simulink model "InverterTestSystemMotorSettings_168_124"  (R2020a)
settings: Solver=ode4  StartTime=0.0  StopTime=inf  FixedStep=Ts  RelTol=1e-3  EnableMultiTasking=on
values from neighbouring files (symbols this model uses):
  SimulinkOutputBusChannelCount = c    [ITS_Create_Simulation_Interface_Buses.m]
undefined symbols (not defined in the file or in its folder): DiscIntNeverNeededParam, signal1, signal2, signal3, signal4, signal5, signal6, signal7
settings Model: SimulationMode=external  ExtModeTrigDuration=16000  ExtModeTrigLevel=10  Creator=Vincent  LastModifiedBy=maccl
settings SolverCC: PositivePriorityOrder=on  AutoInsertRateTranBlk=on  InsertRTBMode=Always
settings DataIOCC: LimitDataPoints=on  MaxDataPoints=200000  SaveFormat=Array  SaveOutput=off  SignalLogging=off  DSMLogging=off  SaveTime=off  ReturnWorkspaceOutputs=off
settings OptimizationCC: EnhancedBackFolding=on  PassReuseOutputArgsThreshold=0  ExpressionDepthLimit=2147483647  LifeSpan=1095  MaxStackSize=64  OptimizeBlockOrder=speed  DifferentSizesBufferReuse=on  OptimizationCustomize=off
settings DebuggingCC: UnderspecifiedInitializationDetection=Classic  MergeDetectMultiDrivingBlocksExec=none  SolverPrmCheckMsg=warning  ParameterTunabilityLossMsg=error  BusObjectLabelMismatch=none  StateNameClashWarn=warning  SFUnexpectedBacktrackingDiag=warning  SFNoUnconditionalDefaultTransitionDiag=warning  SFExecutionAtInitializationDiag=none  ArithmeticOperatorsInVariantConditions=warning
settings HardwareCC: ProdBitPerLong=64  ProdHWDeviceType=Intel->x86-64 (Linux 64)  TargetHWDeviceType=32-bit Generic
settings SFSimCC: SimUseLocalCustomCode=off  CustomCodeUndefinedFunction=UseInterfaceOnly
settings RTWCC: Description=slxrt NI Linux Real-Time x86_64 Targets  SystemTargetFile=ni_slxrt.tlc  PackageName=main_code.zip  GenerateReport=on  RTWUseLocalCustomCode=off  Toolchain=GCC Compiler for VeriStand NI Linux Real-Time targets | gmake makefile (64-bit Windows)  BuildConfiguration=Faster Runs  LaunchReport=on
settings CodeAppCC: ForceParamTrailComments=on  OperatorAnnotations=on  MATLABSourceComments=on
settings STFCustomTargetCC: UseToolchainInfoCompliant=on  SystemTargetFile=ni_slxrt.tlc
settings GRTTargetCC: TargetLangStandard=C89/C90 (ANSI)  ParMdlRefBuildCompliant=off  CompOptLevelCompliant=off  ConcurrentExecutionCompliant=off  CombineOutputUpdateFcns=off  MatFileLogging=off  CPPClassGenCompliant=off  ExtMode=on  ExtModeMexArgs='10.0.35.12',0,17725  RTWCAPISignals=on  RTWCAPIParams=on  RTWCAPIStates=on  RTWCAPIRootIO=on
settings ConfigComp: CovMetricSettings=dw  CovHtmlReporting=on  CovSaveCumulativeToWorkspaceVar=on  CovSaveSingleToWorkspaceVar=on  CovExternalEMLEnable=off

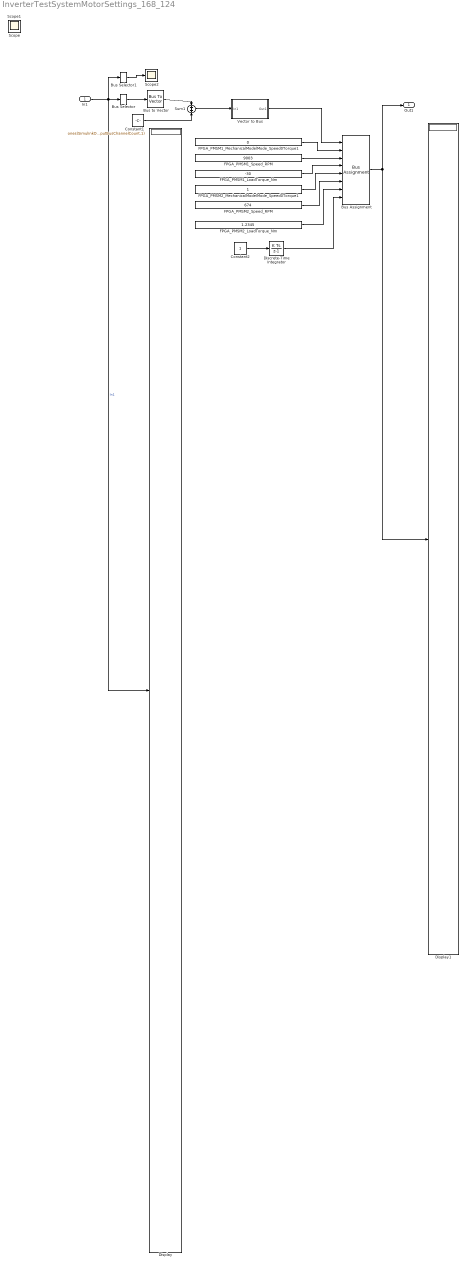
== system InverterTestSystemMotorSettings_168_124 ==
  In1 : Inport  OutDataTypeStr=Bus: SimulinkInputBus
  Bus Assignment : BusAssignment  AssignedSignals=signal1,signal2,signal3,signal4,signal5,signal6,signal7
  Bus Selector : BusSelector  OutputSignals=In001_PMSM1_CurrentPhaseA_A,In002_PMSM1_CurrentPhaseB_A,In003_PMSM1_CurrentPhaseC_A,In004_PMSM1_VoltageAveragePhaseA_V,In005_PMSM1_VoltageAveragePhaseB_V,In006_PMSM1_VoltageAveragePhaseC_V,In007_PMSM1_ThreePhaseActivePower_W,In008_PMSM1_ThreePhaseReactivePower_VAR,In009_PMSM1_DirectStatorCurrentId_A,In010_PMSM1_QuadratureStatorCurrentIq_A,In011_PMSM1_MechanicalAngle_deg,In012_PMSM1_ElectricalAngle_deg,In013_PMSM1_Torque_Nm,In014_PMSM1_ResolverSine,In015_PMSM1_ResolverCosine,In016_PMSM1_ResolverCarrier,In017_PMSM1_ResolverAngle_deg,In018_PMSM1_Speed_RPM,In019_PMSM1_TotalTorque_Nm,In020_PMSM1_BackEMFPhaseA_V,In021_PMSM1_BackEMFPhaseB_V,In022_PMSM1_BackEMFPhaseC_V,In023_PMSM2_CurrentPhaseA_A,In024_PMSM2_CurrentPhaseB_A,In025_PMSM2_CurrentPhaseC_A,In026_PMSM2_VoltageAveragePhaseA_V,In027_PMSM2_VoltageAveragePhaseB_V,In028_PMSM2_VoltageAveragePhaseC_V,In029_PMSM2_ThreePhaseActivePower_W,In030_PMSM2_ThreePhaseReactivePower_VAR,In031_PMSM2_DirectStatorCurrentId_A,In032_PMSM2_QuadratureStatorCurrentIq_A,In033_PMSM2_MechanicalAngle_deg,In034_PMSM2_ElectricalAngle_deg,In035_PMSM2_Torque_Nm,In036_PMSM2_ResolverSine,In037_PMSM2_ResolverCosine,In038_PMSM2_ResolverCarrier,In039_PMSM2_ResolverAngle_deg,In040_PMSM2_Speed_RPM,In041_PMSM2_TotalTorque_Nm,In042_PMSM2_BackEMFPhaseA_V,In043_PMSM2_BackEMFPhaseB_V,In044_PMSM2_BackEMFPhaseC_V,In045_Measurements_001,In046_Measurements_002,In047_Measurements_003,In048_Measurements_004,In049_Measurements_005,In050_Measurements_006,In051_Measurements_007,In052_Measurements_008,In053_Measurements_009,In054_Measurements_010,In055_Measurements_011,In056_Measurements_012,In057_Measurements_013,In058_Measurements_014,In059_Measurements_015,In060_Measurements_016,In061_Measurements_017,In062_Measurements_018,In063_Measurements_019,In064_Measurements_020,In065_Measurements_021,In066_Measurements_022,In067_Measurements_023,In068_Measurements_024,In069_Measurements_025,In070_Measurements_026,In071_Measurements_027,In072_Measurements_028,In073_Measurements_029,In074_Measurements_030,In075_Measurements_031,In076_Measurements_032,In077_Measurements_033,In078_Measurements_034,In079_Measurements_035,In080_Measurements_036,In081_Measurements_037,In082_Measurements_038,In083_Measurements_039,In084_Measurements_040,In085_Measurements_041,In086_Measurements_042,In087_Measurements_043,In088_Measurements_044,In089_Measurements_045,In090_Measurements_046,In091_Measurements_047,In092_Measurements_048,In093_Measurements_049,In094_Measurements_050,In095_Measurements_051,In096_Measurements_052,In097_Measurements_053,In098_Measurements_054,In099_Measurements_055,In100_Measurements_056,In101_Measurements_057,In102_Measurements_058,In103_Measurements_059,In104_Measurements_060,In105_Measurements_061,In106_Measurements_062,In107_Measurements_063,In108_Measurements_064,In109_AnalogOutputs_001,In110_AnalogOutputs_002,In111_AnalogOutputs_003,In112_AnalogOutputs_004,In113_AnalogOutputs_005,In114_AnalogOutputs_006,In115_AnalogOutputs_007,In116_AnalogOutputs_008,In117_AnalogOutputs_009,In118_AnalogOutputs_010,In119_AnalogOutputs_011,In120_AnalogOutputs_012,In121_AnalogOutputs_013,In122_AnalogOutputs_014,In123_AnalogOutputs_015,In124_AnalogOutputs_016  OutputAsBus=on
  Bus Selector1 : BusSelector  OutputSignals=In001_PMSM1_CurrentPhaseA_A,In002_PMSM1_CurrentPhaseB_A,In003_PMSM1_CurrentPhaseC_A  OutputAsBus=on
  Bus to Vector : BusToVector
  Constant1 : Constant  Value=ones(SimulinkOutputBusChannelCount,1)  SampleTime=-1
  Constant2 : Constant  SampleTime=-1
  Discrete-Time Integrator : DiscreteIntegrator  SampleTime=-1  ICPrevOutput=DiscIntNeverNeededParam  ICPrevScaledInput=DiscIntNeverNeededParam
  Display : Display
  Display1 : Display
  FPGA_PMSM1_LoadTorque_Nm : Constant  Value=-30  SampleTime=-1
  FPGA_PMSM1_MechanicalModelMode_Speed0Torque1 : Constant  Value=0  SampleTime=-1
  FPGA_PMSM1_Speed_RPM : Constant  Value=9003  SampleTime=-1
  FPGA_PMSM2_LoadTorque_Nm : Constant  Value=1.2345  SampleTime=-1
  FPGA_PMSM2_MechanicalModelMode_Speed0Torque1 : Constant  SampleTime=-1
  FPGA_PMSM2_Speed_RPM : Constant  Value=674  SampleTime=-1
  Scope2 : Scope
  Sum1 : Sum
  Vector to Bus : Subsystem  mask{Nsigs=SimulinkOutputBusChannelCount}
      mask prompts: Nsigs "Signal Length"
      mask init:
      | CurrentSys = gcs;
      | blockName = get_param(gcb,'Name');
      | oldNsigs = str2num(get_param([CurrentSys '/' blockName '/Demux'],'Outputs'));
      | newNsigs = str2num(get_param([CurrentSys '/' blockName], 'Nsigs'));
      | 
      | if newNsigs > oldNsigs,
      |     set_param([CurrentSys '/' blockName '/Demux'],'Outputs',num2str(newNsigs))
      |     set_param([CurrentSys '/' blockName '/BusCreator'],'Inputs',num2str(newNsigs))
      |     for nnn = (oldNsigs+1):newNsigs,
      |         add_line([CurrentSys '/' blockName],['Demux/' num2str(nnn)],['BusCreator/' num2str(nnn)])
      |     end
      | elseif newNsigs < oldNsigs,
      |     for nnn = (newNsigs+1):oldNsigs,
      |         delete_line([CurrentSys '/' blockName],['Demux/' num2str(nnn)],['BusCreator/' num2str(nnn)])
      |     end
      |     set_param([CurrentSys '/' blockName '/Demux'],'Outputs',num2str(newNsigs))
      |     set_param([CurrentSys '/' blockName '/BusCreator'],'Inputs',num2str(newNsigs))
      | end
  Out1 : Outport  SignalName=Out1  OutDataTypeStr=Bus: SimulinkOutputBus  VectorParamsAs1DForOutWhenUnconnected=off
  Scope : Scope
  Scope1 : Scope
  wires:
  In1/1 -> Bus Selector1/1, Bus Selector/1, Display/1  "In1"
  Constant1/1 -> Sum1/2
  Bus to Vector/1 -> Sum1/1
  Sum1/1 -> Vector to Bus/1(In1)
  Bus Selector/1 -> Bus to Vector/1
  Vector to Bus/1(Out1) -> Bus Assignment/1
  Bus Assignment/1 -> Out1/1, Display1/1
  FPGA_PMSM1_MechanicalModelMode_Speed0Torque1/1 -> Bus Assignment/2
  FPGA_PMSM1_Speed_RPM/1 -> Bus Assignment/3
  FPGA_PMSM1_LoadTorque_Nm/1 -> Bus Assignment/4
  FPGA_PMSM2_MechanicalModelMode_Speed0Torque1/1 -> Bus Assignment/5
  FPGA_PMSM2_Speed_RPM/1 -> Bus Assignment/6
  FPGA_PMSM2_LoadTorque_Nm/1 -> Bus Assignment/7
  Constant2/1 -> Discrete-Time Integrator/1
  Discrete-Time Integrator/1 -> Bus Assignment/8
  Bus Selector1/1 -> Scope2/1

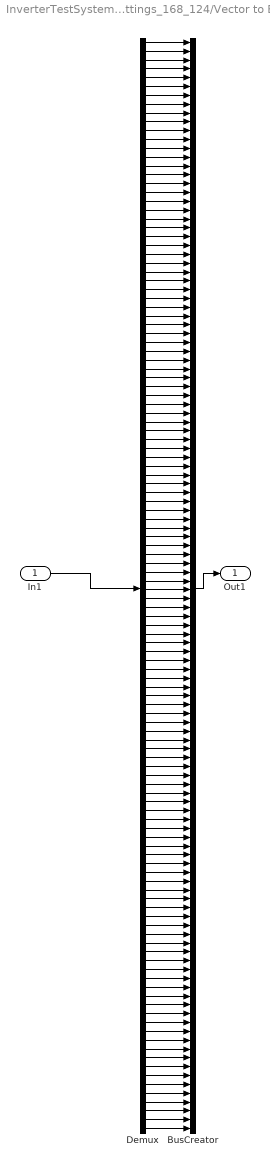
== system InverterTestSystemMotorSettings_168_124/Vector to Bus ==
  In1 : Inport
  BusCreator : BusCreator  Inputs=124
  Demux : Demux  Outputs=124
  Out1 : Outport  VectorParamsAs1DForOutWhenUnconnected=off
  wires:
  Demux/7 -> BusCreator/7
  Demux/6 -> BusCreator/6
  Demux/5 -> BusCreator/5
  Demux/1 -> BusCreator/1
  Demux/2 -> BusCreator/2
  BusCreator/1 -> Out1/1
  In1/1 -> Demux/1
  Demux/3 -> BusCreator/3
  Demux/4 -> BusCreator/4
  Demux/8 -> BusCreator/8
  Demux/9 -> BusCreator/9
  Demux/10 -> BusCreator/10
  Demux/11 -> BusCreator/11
  Demux/12 -> BusCreator/12
  Demux/13 -> BusCreator/13
  Demux/14 -> BusCreator/14
  Demux/15 -> BusCreator/15
  Demux/16 -> BusCreator/16
  Demux/17 -> BusCreator/17
  Demux/18 -> BusCreator/18
  Demux/19 -> BusCreator/19
  Demux/20 -> BusCreator/20
  Demux/21 -> BusCreator/21
  Demux/22 -> BusCreator/22
  Demux/23 -> BusCreator/23
  Demux/24 -> BusCreator/24
  Demux/25 -> BusCreator/25
  Demux/26 -> BusCreator/26
  Demux/27 -> BusCreator/27
  Demux/28 -> BusCreator/28
  Demux/29 -> BusCreator/29
  Demux/30 -> BusCreator/30
  Demux/31 -> BusCreator/31
  Demux/32 -> BusCreator/32
  Demux/33 -> BusCreator/33
  Demux/34 -> BusCreator/34
  Demux/35 -> BusCreator/35
  Demux/36 -> BusCreator/36
  Demux/37 -> BusCreator/37
  Demux/38 -> BusCreator/38
  Demux/39 -> BusCreator/39
  Demux/40 -> BusCreator/40
  Demux/41 -> BusCreator/41
  Demux/42 -> BusCreator/42
  Demux/43 -> BusCreator/43
  Demux/44 -> BusCreator/44
  Demux/45 -> BusCreator/45
  Demux/46 -> BusCreator/46
  Demux/47 -> BusCreator/47
  Demux/48 -> BusCreator/48
  Demux/49 -> BusCreator/49
  Demux/50 -> BusCreator/50
  Demux/51 -> BusCreator/51
  Demux/52 -> BusCreator/52
  Demux/53 -> BusCreator/53
  Demux/54 -> BusCreator/54
  Demux/55 -> BusCreator/55
  Demux/56 -> BusCreator/56
  Demux/57 -> BusCreator/57
  Demux/58 -> BusCreator/58
  Demux/59 -> BusCreator/59
  Demux/60 -> BusCreator/60
  Demux/61 -> BusCreator/61
  Demux/62 -> BusCreator/62
  Demux/63 -> BusCreator/63
  Demux/64 -> BusCreator/64
  Demux/65 -> BusCreator/65
  Demux/66 -> BusCreator/66
  Demux/67 -> BusCreator/67
  Demux/68 -> BusCreator/68
  Demux/69 -> BusCreator/69
  Demux/70 -> BusCreator/70
  Demux/71 -> BusCreator/71
  Demux/72 -> BusCreator/72
  Demux/73 -> BusCreator/73
  Demux/74 -> BusCreator/74
  Demux/75 -> BusCreator/75
  Demux/76 -> BusCreator/76
  Demux/77 -> BusCreator/77
  Demux/78 -> BusCreator/78
  Demux/79 -> BusCreator/79
  Demux/80 -> BusCreator/80
  Demux/81 -> BusCreator/81
  Demux/82 -> BusCreator/82
  Demux/83 -> BusCreator/83
  Demux/84 -> BusCreator/84
  Demux/85 -> BusCreator/85
  Demux/86 -> BusCreator/86
  Demux/87 -> BusCreator/87
  Demux/88 -> BusCreator/88
  Demux/89 -> BusCreator/89
  Demux/90 -> BusCreator/90
  Demux/91 -> BusCreator/91
  Demux/92 -> BusCreator/92
  Demux/93 -> BusCreator/93
  Demux/94 -> BusCreator/94
  Demux/95 -> BusCreator/95
  Demux/96 -> BusCreator/96
  Demux/97 -> BusCreator/97
  Demux/98 -> BusCreator/98
  Demux/99 -> BusCreator/99
  Demux/100 -> BusCreator/100
  Demux/101 -> BusCreator/101
  Demux/102 -> BusCreator/102
  Demux/103 -> BusCreator/103
  Demux/104 -> BusCreator/104
  Demux/105 -> BusCreator/105
  Demux/106 -> BusCreator/106
  Demux/107 -> BusCreator/107
  Demux/108 -> BusCreator/108
  Demux/109 -> BusCreator/109
  Demux/110 -> BusCreator/110
  Demux/111 -> BusCreator/111
  Demux/112 -> BusCreator/112
  Demux/113 -> BusCreator/113
  Demux/114 -> BusCreator/114
  Demux/115 -> BusCreator/115
  Demux/116 -> BusCreator/116
  Demux/117 -> BusCreator/117
  Demux/118 -> BusCreator/118
  Demux/119 -> BusCreator/119
  Demux/120 -> BusCreator/120
  Demux/121 -> BusCreator/121
  Demux/122 -> BusCreator/122
  Demux/123 -> BusCreator/123
  Demux/124 -> BusCreator/124
